simulink model "task2Model"  (Simulink 7.5)
settings: Solver=ode3  StartTime=0.0  StopTime=300  FixedStep=1  RelTol=1e-3
undefined symbols (not defined in the file): DiscIntNeverNeededParam
settings Model: Creator=Dranik_win  LastModifiedBy=Dranik_win
settings SimEventsCC: propDiagAttribOutput=1  propDiagFcnCallOutput=1  propDiagStatOutput=0

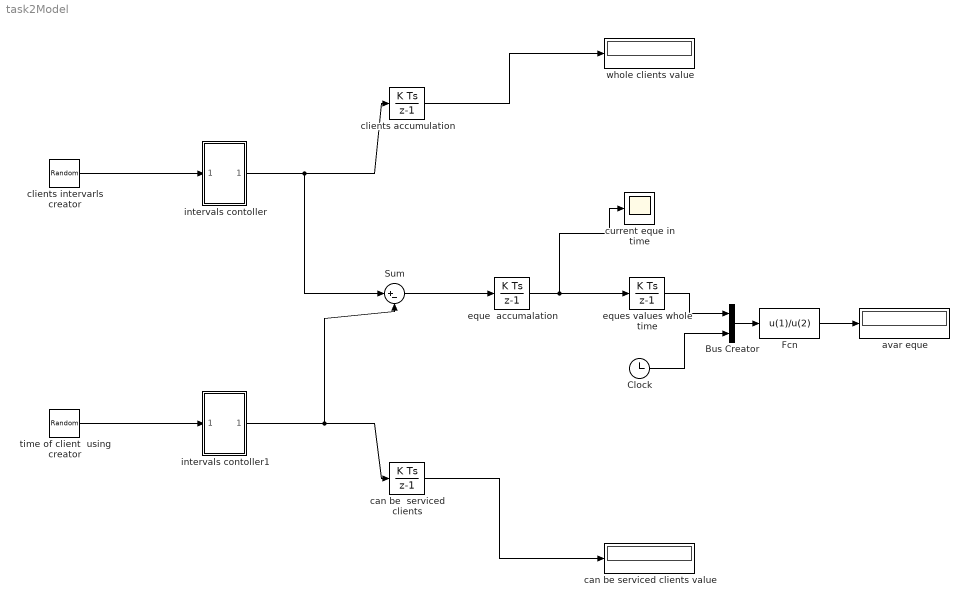
== system task2Model ==
  Bus Creator : BusCreator  Inputs=2
  Clock : Clock
      settings: Decimation=10
  Fcn : Fcn  Expr=u(1)/u(2)
  Sum : Sum  Inputs=|+-  OutDataType=fixdt(1, 16)  OutScaling=2^0
  avar eque : Display
  can be  serviced clients : DiscreteIntegrator  OutDataType=fixdt(1, 16)  OutScaling=2^0  ICPrevOutput=DiscIntNeverNeededParam  ICPrevScaledInput=DiscIntNeverNeededParam
  can be serviced clients value : Display
  clients accumulation : DiscreteIntegrator  OutDataType=fixdt(1, 16)  OutScaling=2^0  ICPrevOutput=DiscIntNeverNeededParam  ICPrevScaledInput=DiscIntNeverNeededParam
  clients intervarls creator : RandomNumber  Mean=10  Variance=4
  current eque in time : Scope
  eque  accumalation : DiscreteIntegrator  OutDataType=fixdt(1, 16)  OutScaling=2^0  LimitOutput=on  LowerSaturationLimit=0  ICPrevOutput=DiscIntNeverNeededParam  ICPrevScaledInput=DiscIntNeverNeededParam
  eques values whole time : DiscreteIntegrator  OutDataType=fixdt(1, 16)  OutScaling=2^0  ICPrevOutput=DiscIntNeverNeededParam  ICPrevScaledInput=DiscIntNeverNeededParam
  intervals contoller : Subsystem
  intervals contoller1 : Subsystem
  time of client  using creator : RandomNumber  Mean=7  Variance=4
  whole clients value : Display
  wires:
  clients intervarls creator/1 -> intervals contoller/1(In1)
  intervals contoller/1(Out1) -> clients accumulation/1, Sum/1
  clients accumulation/1 -> whole clients value/1
  time of client  using creator/1 -> intervals contoller1/1(In1)
  intervals contoller1/1(Out1) -> can be  serviced clients/1, Sum/2
  can be  serviced clients/1 -> can be serviced clients value/1
  Sum/1 -> eque  accumalation/1
  eque  accumalation/1 -> current eque in time/1, eques values whole time/1
  eques values whole time/1 -> Bus Creator/1
  Clock/1 -> Bus Creator/2
  Bus Creator/1 -> Fcn/1
  Fcn/1 -> avar eque/1

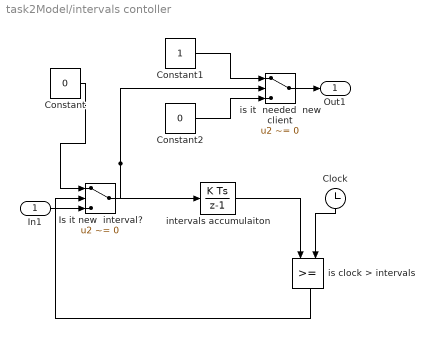
== system task2Model/intervals contoller ==
  In1 : Inport
  Clock : Clock
      settings: Decimation=10
  Constant : Constant  Value=0  OutDataType=fixdt(1, 16)  OutScaling=2^0
  Constant1 : Constant  OutDataType=fixdt(1, 16)  OutScaling=2^0
  Constant2 : Constant  Value=0  OutDataType=fixdt(1, 16)  OutScaling=2^0
  Is it new  interval? : Switch  Criteria=u2 ~= 0  OutDataType=fixdt(1, 16)  OutScaling=2^0
  intervals accumulaiton : DiscreteIntegrator  OutDataType=fixdt(1, 16)  OutScaling=2^0  ICPrevOutput=DiscIntNeverNeededParam  ICPrevScaledInput=DiscIntNeverNeededParam
  is clock > intervals : RelationalOperator  LogicOutDataTypeMode=boolean  LogicDataType=fixdt(0, 8)  OutDataTypeStr=boolean
  is it  needed  new client : Switch  Criteria=u2 ~= 0  OutDataType=fixdt(1, 16)  OutScaling=2^0
  Out1 : Outport
  wires:
  Constant1/1 -> is it  needed  new client/1
  Constant2/1 -> is it  needed  new client/3
  Constant/1 -> Is it new  interval?/1
  Is it new  interval?/1 -> intervals accumulaiton/1, is it  needed  new client/2
  is clock > intervals/1 -> Is it new  interval?/2
  Clock/1 -> is clock > intervals/2
  intervals accumulaiton/1 -> is clock > intervals/1
  is it  needed  new client/1 -> Out1/1
  In1/1 -> Is it new  interval?/3

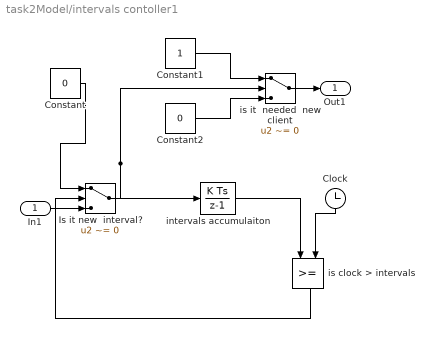
== system task2Model/intervals contoller1 ==
  In1 : Inport
  Clock : Clock
      settings: Decimation=10
  Constant : Constant  Value=0  OutDataType=fixdt(1, 16)  OutScaling=2^0
  Constant1 : Constant  OutDataType=fixdt(1, 16)  OutScaling=2^0
  Constant2 : Constant  Value=0  OutDataType=fixdt(1, 16)  OutScaling=2^0
  Is it new  interval? : Switch  Criteria=u2 ~= 0  OutDataType=fixdt(1, 16)  OutScaling=2^0
  intervals accumulaiton : DiscreteIntegrator  OutDataType=fixdt(1, 16)  OutScaling=2^0  ICPrevOutput=DiscIntNeverNeededParam  ICPrevScaledInput=DiscIntNeverNeededParam
  is clock > intervals : RelationalOperator  LogicOutDataTypeMode=boolean  LogicDataType=fixdt(0, 8)  OutDataTypeStr=boolean
  is it  needed  new client : Switch  Criteria=u2 ~= 0  OutDataType=fixdt(1, 16)  OutScaling=2^0
  Out1 : Outport
  wires:
  Constant1/1 -> is it  needed  new client/1
  Constant2/1 -> is it  needed  new client/3
  Constant/1 -> Is it new  interval?/1
  Is it new  interval?/1 -> intervals accumulaiton/1, is it  needed  new client/2
  is clock > intervals/1 -> Is it new  interval?/2
  Clock/1 -> is clock > intervals/2
  intervals accumulaiton/1 -> is clock > intervals/1
  is it  needed  new client/1 -> Out1/1
  In1/1 -> Is it new  interval?/3
